simulink model "Regler_Loop_hard"  (R2025b)
settings: Solver=ode23s  StartTime=tSim(1)  StopTime=tSim(end)  FixedStep=tStep  RelTol=1e-3  EnableMultiTasking=on
values from neighbouring files (symbols this model uses):
  M_max = 0.4    [reglerInit.m]
settings Model: Creator=Henning Schlüter  LastModifiedBy=fabim
settings SolverCC: AlgebraicLoopSolver=TrustRegion
settings DataIOCC: SaveFormat=Array  SignalLoggingSaveFormat=ModelDataLogs  SaveOutput=off  SaveTime=off  ReturnWorkspaceOutputs=off
settings OptimizationCC: ExpressionDepthLimit=2147483647.0  LifeSpan=inf
settings DebuggingCC: UnderspecifiedInitializationDetection=Classic  MergeDetectMultiDrivingBlocksExec=none  SolverPrmCheckMsg=warning  UnconnectedInputMsg=warning  UnconnectedOutputMsg=warning  UnconnectedLineMsg=warning  StateNameClashWarn=warning  PregeneratedLibrarySubsystemCodeDiagnostic=none  SFUnexpectedBacktrackingDiag=warning  SFNoUnconditionalDefaultTransitionDiag=warning  SFExecutionAtInitializationDiag=none  ArithmeticOperatorsInVariantConditions=warning
settings HardwareCC: ProdBitPerPointer=32.0  ProdBitPerSizeT=32.0  ProdBitPerPtrDiffT=32.0  ProdLargestAtomicFloat=None  ProdIntDivRoundTo=Undefined  ProdEndianess=Unspecified  ProdWordSize=32.0  ProdHWDeviceType=32-bit Generic
settings ModelReferenceCC: EnableRefExpFcnMdlSchedulingChecks=on  PropagateSignalLabelsOutOfModel=off
settings SFSimCC: SimUseLocalCustomCode=off  CustomCodeUndefinedFunction=UseInterfaceOnly
settings RTWCC: RTWUseLocalCustomCode=off  GPUComputeCapability=3.5
settings CodeAppCC: StateflowObjectComments=on
settings GRTTargetCC: TargetLangStandard=C89/C90 (ANSI)  CombineOutputUpdateFcns=off  GRTInterface=on
settings ConfigComp: CovMetricSettings=dw  CovSaveCumulativeToWorkspaceVar=on  CovSaveSingleToWorkspaceVar=on  CovExternalEMLEnable=off  CovSFcnEnable=off

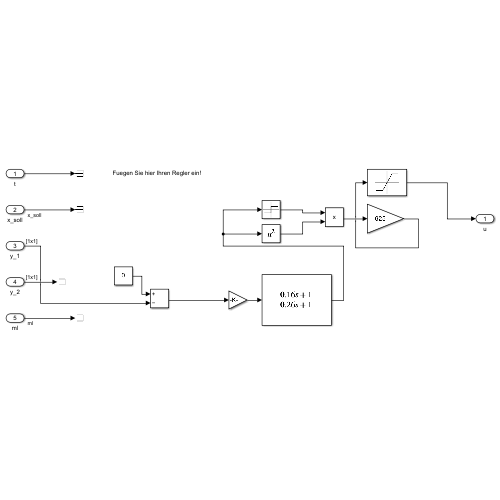
[thumbnail: Simulink's stored preview of the top-level diagram]
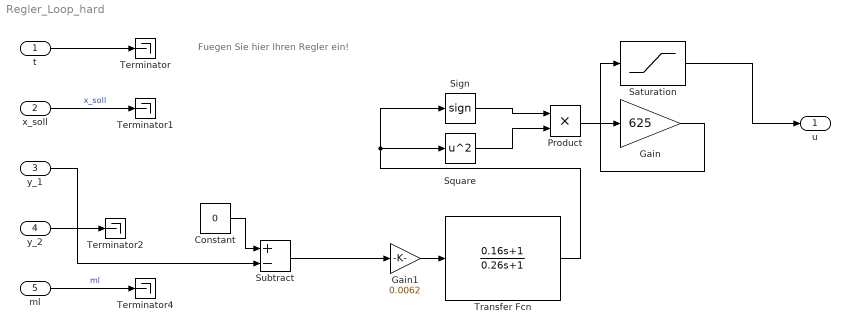
== system Regler_Loop_hard ==
  note: Fuegen Sie hier Ihren Regler ein!
  t : Inport  OutDataTypeStr=double  PortDimensions=1  SampleTime=0
  "x_soll " : Inport  Port=2  OutDataTypeStr=double  PortDimensions=1  SampleTime=0
  y_1 : Inport  Port=3  OutDataTypeStr=double  PortDimensions=[1 1]  SampleTime=0
  y_2 : Inport  Port=4  OutDataTypeStr=double  PortDimensions=[1 1]  SampleTime=0
  ml : Inport  Port=5  OutDataTypeStr=double  PortDimensions=1  SampleTime=0
  Constant : Constant  Value=0
  Gain : Gain  Gain=625
  Gain1 : Gain  Gain=0.0062
  Product : Product
  Saturation : Saturate  UpperLimit=M_max  LowerLimit=-M_max
  Sign : Signum
  Square : Math  Operator=square
  Subtract : Sum  Inputs=+-
  Terminator{,1..2,4} (4 alike) : Terminator
  Transfer Fcn : TransferFcn  Numerator=[0.16 1]  Denominator=[0.26 1]
  u : Outport  OutDataTypeStr=double  PortDimensions=1  VectorParamsAs1DForOutWhenUnconnected=off
  wires:
  t/1 -> Terminator/1
  "x_soll "/1 -> Terminator1/1  "x_soll"
  ml/1 -> Terminator4/1  "ml"
  Product/1 -> Gain/1
  Square/1 -> Product/2
  Sign/1 -> Product/1
  Gain/1 -> Saturation/1
  Transfer Fcn/1 -> Sign/1, Square/1
  Gain1/1 -> Transfer Fcn/1
  Saturation/1 -> u/1
  Subtract/1 -> Gain1/1
  Constant/1 -> Subtract/1
  y_1/1 -> Subtract/2
  y_2/1 -> Terminator2/1
